simulink model "phxex_sim_stand"  (R2026a)
settings: Solver=VariableStepAuto
libraries: PhxLibrary x1
settings Model: Creator=lzhan  LastModifiedBy=lzhan

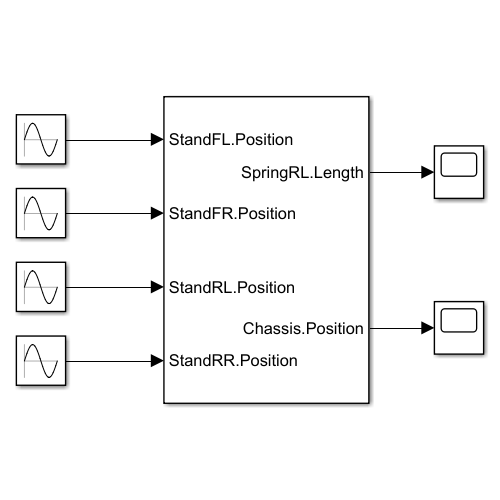
[thumbnail: Simulink's stored preview of the top-level diagram]
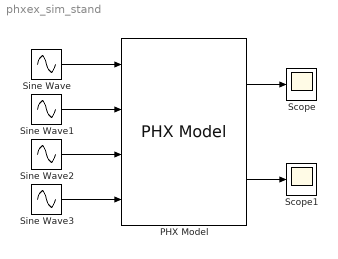
== system phxex_sim_stand ==
  PHX Model : PhxLibrary/PHX Model  ModelSource=saved_stand.mat  InputRefs=|  OutputRefs=|  ShowViewer=on  RenderEach=on  CameraPosition=[-30,-30,30]  CameraTarget=[0,0,0]  SimulationStep=0.01  SimpleIcon=off  Substeps=1  CameraResolution=[0 0]
      InputRefs=|
      | StandFL.Position(3)
      | StandFR.Position(3)
      | StandRL.Position(3)
      | StandRR.Position(3)
      OutputRefs=|
      | SpringRL.Length(1)
      | Chassis.Position
  Scope : Scope
      settings: ActiveDisplayYMinimum=-0.67142714505707235  ActiveDisplayYMaximum=0.094092685046921018
  Scope1 : Scope
      settings: ActiveDisplayYMinimum=-2.0621965890176641  ActiveDisplayYMaximum=12.152547439157718
  Sine Wave : Sin  Amplitude=0.5  Frequency=2*pi  SampleTime=0
  Sine Wave1 : Sin  Amplitude=0.5  Frequency=3*pi  SampleTime=0
  Sine Wave2 : Sin  Amplitude=0.5  Frequency=1.5*pi  SampleTime=0
  Sine Wave3 : Sin  Amplitude=0.5  Frequency=1*pi  SampleTime=0
  wires:
  Sine Wave2/1 -> PHX Model/3
  Sine Wave1/1 -> PHX Model/2
  Sine Wave/1 -> PHX Model/1
  Sine Wave3/1 -> PHX Model/4
  PHX Model/1 -> Scope/1
  PHX Model/2 -> Scope1/1
